simulink model "task_6_model"  (R2020a)
settings: Solver=VariableStepAuto  StartTime=0.0  StopTime=10  RelTol=1e-3
values from neighbouring files (symbols this model uses):
  h = 1    [task_6.m]    (also in task_8.m; task_9.m)
  L = 1    [task_6.m]    (also in task_8.m; task_9.m)
  R = 1    [task_6.m]    (also in task_8.m; task_9.m)
undefined symbols (not defined in the file or in its folder): K
settings Model: Creator=jryl9  LastModifiedBy=jryl9

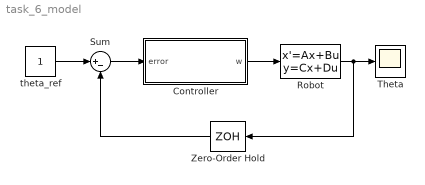
== system task_6_model ==
  Controller : Subsystem
  Robot : StateSpace  A=0  B=R/L  D=0  InitialCondition=0
  Sum : Sum  Inputs=|+-
  Theta : Scope
  Zero-Order Hold : ZeroOrderHold  SampleTime=h
  theta_ref : Constant
  wires:
  Controller/1(w) -> Robot/1
  theta_ref/1 -> Sum/1
  Sum/1 -> Controller/1(error)
  Robot/1 -> Zero-Order Hold/1, Theta/1
  Zero-Order Hold/1 -> Sum/2

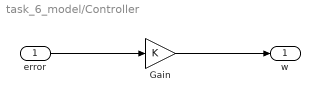
== system task_6_model/Controller ==
  error : Inport
  Gain : Gain  Gain=K
  w : Outport
  wires:
  error/1 -> Gain/1
  Gain/1 -> w/1
